simulink subsystem "PROPAGATOR"  (R2025b)
settings: Solver=VariableStepAuto  StartTime=0.0  StopTime=10.0  RelTol=1e-3
model mask{Parameter10=, Parameter11=, Parameter12=, Parameter13=, Parameter14=, Parameter4=, Parameter5=, Parameter6=, Parameter7=, quatConv=q4 (scalar last), forcesFrame=Inertial, r0=0, v0=0, att0=0, omg0=0, Parameter8=, Parameter9=}
  mask prompts: Parameter10 "State: 13x1 column vector, contains [inertial position; inertial velocity; inertial to body attitude; body to inertial angular velocity], in SI units"; Parameter11 "Force: 3x1 column vector, applied in the vehicle's CoG, in N"; Parameter12 "Torque: 3x1 column vector, applied in the vehicle's CoG, in Nm"; Parameter13 "Mass: 1x1 scalar, total mass of the vehicle, in kg"; Parameter14 "Inertia: 3x3 matrix, inertia tensor of the vehicle, in kgm2"; Parameter4 "Initial position: 3x1 column vector, inertial frame"; Parameter5 "Initial velocity: 3x1 column vector, inertial frame"; Parameter6 "Initial attitude: 4x1 column vector, rotation quaternion from inertial to body"; Parameter7 "Initial angular velocity: 3x1 column vector, angular rates in body frame w.r.t inertial frame"; quatConv "Quaternion convention"; forcesFrame "Forces reference frame"; r0 "Initial position [m]"; v0 "Initial velocity [ms-1]"; att0 "Initial attitude from inertial to body [-]"; omg0 "Initial angular velocity [rads-1]"; Parameter8 "Quaternion convention: Position of the scalar term"; Parameter9 "Forces reference frame: Forces in inertial frame or body frame"
libraries: aerolibutil x2, sharedutil x1, matrix_library x1
settings Model: Creator=antoniohernandez-rodiciomateos  LastModifiedBy=antoniohernandez-rodiciomateos

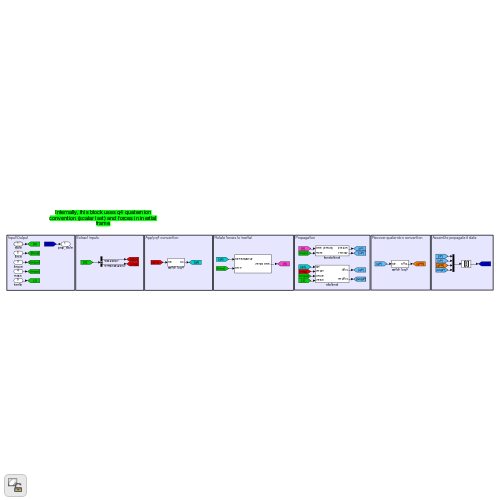
[thumbnail: Simulink's stored preview of the top-level diagram]
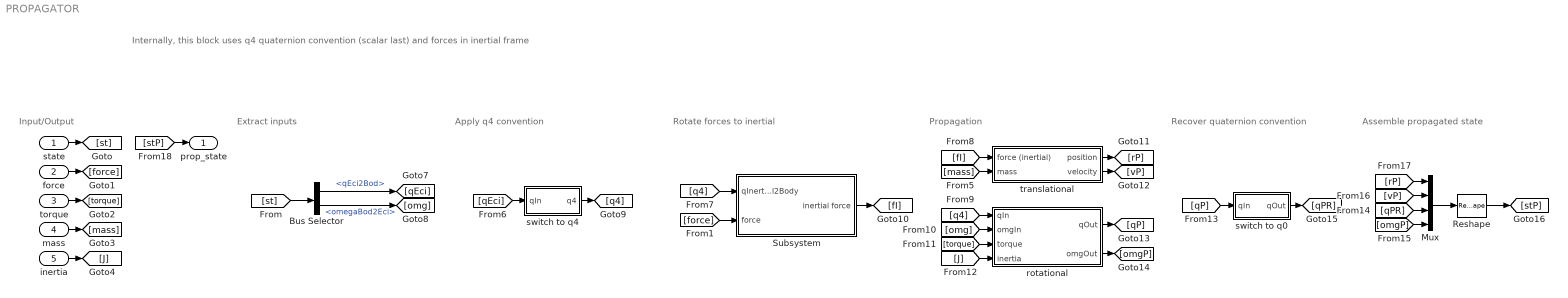
== system PROPAGATOR ==
  note: Input/Output
  note: Internally, this block uses q4 quaternion convention (scalar last) and forces in inertial frame
  note: Extract inputs
  note: Apply q4 convention
  note: Rotate forces to inertial
  note: Propagation
  note: Recover quaternion convention
  note: Assemble propagated state
  state : Inport  OutDataTypeStr=Bus: state_bus  PortDimensions=[13 1]
  force : Inport  Port=2  PortDimensions=[3 1]
  torque : Inport  Port=3  PortDimensions=[3 1]
  mass : Inport  Port=4  PortDimensions=[1 1]
  inertia : Inport  Port=5  PortDimensions=[3 3]
  Bus Selector : BusSelector  OutputSignals=qEci2Bod,omegaBod2Eci
  Mux : Mux
  Reshape : Reshape  OutputDimensionality=Column vector (2-D)
  Subsystem : Subsystem
  rotational : Subsystem
  switch to q0 : Subsystem
  switch to q4 : Subsystem
  translational : Subsystem
  prop_state : Outport  PortDimensions=[13 1]
  wires:
  state/1 -> [st]
  force/1 -> [force]
  torque/1 -> [torque]
  inertia/1 -> [J]
  mass/1 -> [mass]
  [st] -> Bus Selector/1
  Bus Selector/1 -> [qEci]  "<qEci2Bod>"
  Bus Selector/2 -> [omg]  "<omegaBod2Eci>"
  [q4] -> Subsystem/1(qInertial2Body)
  [force] -> Subsystem/2(force)
  [mass] -> translational/2(mass)
  Subsystem/1(inertial force) -> [fI]
  [fI] -> translational/1(force (inertial))
  [q4] -> rotational/1(qIn)
  [omg] -> rotational/2(omgIn)
  [torque] -> rotational/3(torque)
  [J] -> rotational/4(inertia)
  translational/1(position) -> [rP]
  translational/2(velocity) -> [vP]
  rotational/1(qOut) -> [qP]
  rotational/2(omgOut) -> [omgP]
  [qEci] -> switch to q4/1(qIn)
  switch to q4/1(q4) -> [q4]
  [qP] -> switch to q0/1(qIn)
  switch to q0/1(qOut) -> [qPR]
  [qPR] -> Mux/3
  [omgP] -> Mux/4
  [vP] -> Mux/2
  [rP] -> Mux/1
  [stP] -> prop_state/1
  Mux/1 -> Reshape/1
  Reshape/1 -> [stP]

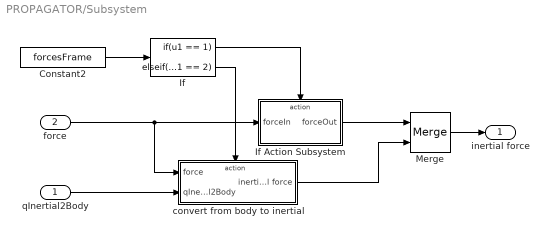
== system PROPAGATOR/Subsystem ==
  qInertial2Body : Inport  PortDimensions=[4 1]
  force : Inport  Port=2  PortDimensions=[3 1]
  Constant2 : Constant  Value=forcesFrame
  If : If  IfExpression=u1 == 1  ElseIfExpressions=u1 == 2  ShowElse=off
  If Action Subsystem : Subsystem  TreatAsAtomicUnit=on
  Merge : Merge
  convert from body to inertial : Subsystem  TreatAsAtomicUnit=on
  inertial force : Outport  PortDimensions=[3 1]
  wires:
  convert from body to inertial/1(inertial force) -> Merge/2
  If/1 -> If Action Subsystem/Action
  If Action Subsystem/1(forceOut) -> Merge/1
  force/1 -> convert from body to inertial/1(force), If Action Subsystem/1(forceIn)
  If/2 -> convert from body to inertial/Action
  Constant2/1 -> If/1
  Merge/1 -> inertial force/1
  qInertial2Body/1 -> convert from body to inertial/2(qInertial2Body)

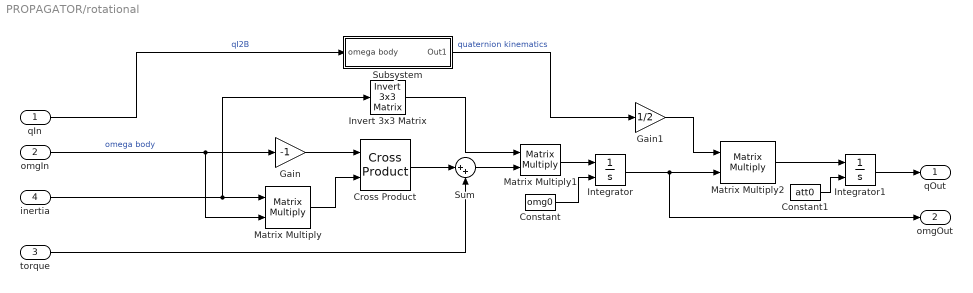
== system PROPAGATOR/rotational ==
  qIn : Inport  PortDimensions=[4 1]
  omgIn : Inport  Port=2  PortDimensions=[3 1]
  torque : Inport  Port=3  PortDimensions=[3 1]
  inertia : Inport  Port=4  PortDimensions=[3 3]
  Constant : Constant  Value=omg0
  Constant1 : Constant  Value=att0
  Cross Product : matrix_library/Cross Product
  Gain : Gain  Gain=-1
  Gain1 : Gain  Gain=1/2
  Integrator : Integrator  InitialConditionSource=external
  Integrator1 : Integrator  InitialConditionSource=external
  Invert 3x3 Matrix : aerolibutil/Invert  3x3 Matrix
  Matrix Multiply : Product  Multiplication=Matrix(*)
  Matrix Multiply1 : Product  Multiplication=Matrix(*)
  Matrix Multiply2 : Product  Multiplication=Matrix(*)
  Subsystem : Subsystem
  Sum : Sum  Inputs=|++
  qOut : Outport  PortDimensions=[4 1]
  omgOut : Outport  Port=2  PortDimensions=[3 1]
  wires:
  inertia/1 -> Invert 3x3 Matrix/1, Matrix Multiply/1
  Matrix Multiply/1 -> Cross Product/2
  omgIn/1 -> Gain/1, Matrix Multiply/2  "omega body"
  Gain/1 -> Cross Product/1
  Cross Product/1 -> Sum/1
  torque/1 -> Sum/2
  Sum/1 -> Matrix Multiply1/2
  Invert 3x3 Matrix/1 -> Matrix Multiply1/1
  Matrix Multiply1/1 -> Integrator/1
  Constant/1 -> Integrator/2
  qIn/1 -> Subsystem/1(omega body)  "qI2B"
  Subsystem/1(Out1) -> Gain1/1  "quaternion kinematics"
  Gain1/1 -> Matrix Multiply2/1
  Integrator/1 -> omgOut/1, Matrix Multiply2/2
  Integrator1/1 -> qOut/1
  Matrix Multiply2/1 -> Integrator1/1
  Constant1/1 -> Integrator1/2

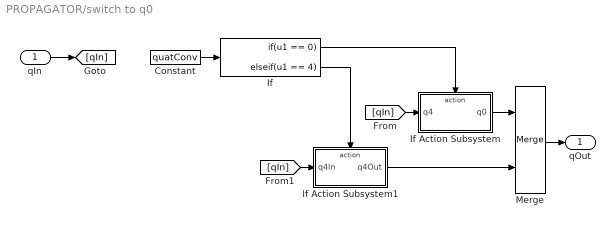
== system PROPAGATOR/switch to q0 ==
  qIn : Inport  PortDimensions=[4 1]
  Constant : Constant  Value=quatConv
  If : If  IfExpression=u1 == 0  ElseIfExpressions=u1 == 4  ShowElse=off
  If Action Subsystem : Subsystem  TreatAsAtomicUnit=on
  If Action Subsystem1 : Subsystem  TreatAsAtomicUnit=on
  Merge : Merge
  qOut : Outport  PortDimensions=[4 1]
  wires:
  If/1 -> If Action Subsystem/Action
  Merge/1 -> qOut/1
  Constant/1 -> If/1
  [qIn] -> If Action Subsystem/1(q4)
  If Action Subsystem1/1(q4Out) -> Merge/2
  [qIn] -> If Action Subsystem1/1(q4In)
  If Action Subsystem/1(q0) -> Merge/1
  If/2 -> If Action Subsystem1/Action
  qIn/1 -> [qIn]

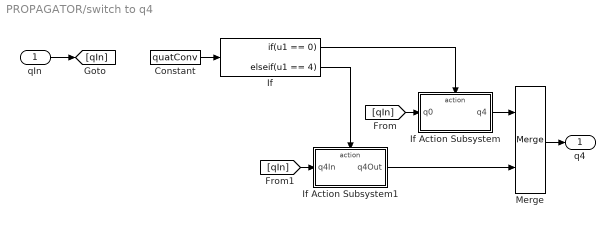
== system PROPAGATOR/switch to q4 ==
  qIn : Inport  PortDimensions=[4 1]
  Constant : Constant  Value=quatConv
  If : If  IfExpression=u1 == 0  ElseIfExpressions=u1 == 4  ShowElse=off
  If Action Subsystem : Subsystem  TreatAsAtomicUnit=on
  If Action Subsystem1 : Subsystem  TreatAsAtomicUnit=on
  Merge : Merge
  q4 : Outport  PortDimensions=[4 1]
  wires:
  If/1 -> If Action Subsystem/Action
  Merge/1 -> q4/1
  Constant/1 -> If/1
  [qIn] -> If Action Subsystem/1(q0)
  If Action Subsystem1/1(q4Out) -> Merge/2
  [qIn] -> If Action Subsystem1/1(q4In)
  If Action Subsystem/1(q4) -> Merge/1
  If/2 -> If Action Subsystem1/Action
  qIn/1 -> [qIn]

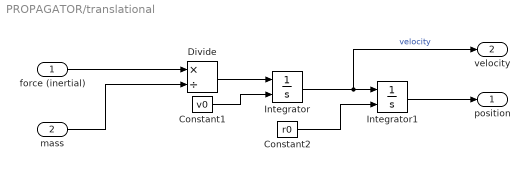
== system PROPAGATOR/translational ==
  force (inertial) : Inport  PortDimensions=[3 1]
  mass : Inport  Port=2  PortDimensions=[1 1]
  Constant1 : Constant  Value=v0
  Constant2 : Constant  Value=r0
  Divide : Product  Inputs=*/
  Integrator : Integrator  InitialConditionSource=external
  Integrator1 : Integrator  InitialConditionSource=external
  position : Outport  PortDimensions=[3 1]
  velocity : Outport  Port=2  PortDimensions=[3 1]
  wires:
  mass/1 -> Divide/2
  Constant1/1 -> Integrator/2
  Constant2/1 -> Integrator1/2
  Divide/1 -> Integrator/1
  Integrator1/1 -> position/1
  force (inertial)/1 -> Divide/1
  Integrator/1 -> velocity/1, Integrator1/1  "velocity"

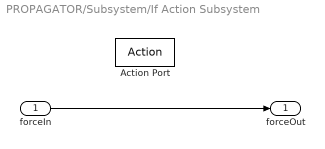
== system PROPAGATOR/Subsystem/If Action Subsystem ==
  forceIn : Inport  PortDimensions=[3 1]
  Action Port : ActionPort
  forceOut : Outport  PortDimensions=[3 1]
  wires:
  forceIn/1 -> forceOut/1

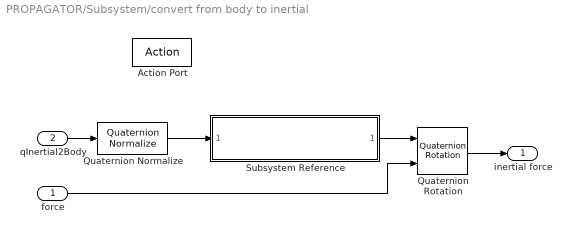
== system PROPAGATOR/Subsystem/convert from body to inertial ==
  force : Inport
  qInertial2Body : Inport  Port=2
  Action Port : ActionPort
  Quaternion Normalize : sharedutil/Quaternion Normalize  aMode=aMode
  Quaternion Rotation : aerolibutil/Quaternion Rotation
  Subsystem Reference : Subsystem  ReferencedSubsystem=quatConventionConverter  conversion=q4 to q0
  inertial force : Outport
  wires:
  force/1 -> Quaternion Rotation/2
  qInertial2Body/1 -> Quaternion Normalize/1
  Quaternion Normalize/1 -> Subsystem Reference/1
  Subsystem Reference/1 -> Quaternion Rotation/1
  Quaternion Rotation/1 -> inertial force/1

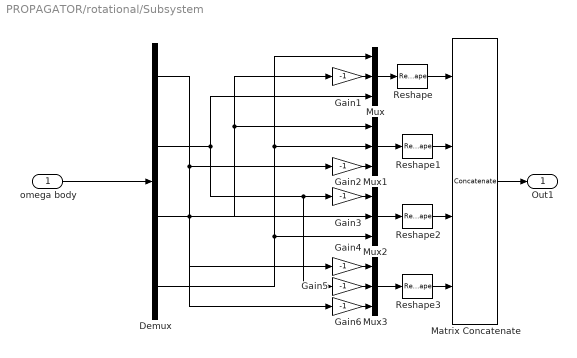
== system PROPAGATOR/rotational/Subsystem ==
  omega body : Inport  PortDimensions=[4 1]
  Demux : Demux
  Gain{1..6} (6 alike) : Gain  Gain=-1
  Matrix Concatenate : Concatenate  NumInputs=4  Mode=Multidimensional array
  Mux{,1..3} (4 alike) : Mux  Inputs=3
  Reshape{,1..3} (4 alike) : Reshape  OutputDimensionality=Row vector (2-D)
  Out1 : Outport  PortDimensions=[4 3]
  wires:
  omega body/1 -> Demux/1
  Mux/1 -> Reshape/1
  Reshape1/1 -> Matrix Concatenate/2
  Mux3/1 -> Reshape3/1
  Matrix Concatenate/1 -> Out1/1
  Reshape2/1 -> Matrix Concatenate/3
  Gain2/1 -> Mux1/3
  Gain5/1 -> Mux3/2
  Reshape3/1 -> Matrix Concatenate/4
  Mux2/1 -> Reshape2/1
  Demux/2 -> Gain5/1, Gain3/1, Mux/3
  Gain3/1 -> Mux2/1
  Demux/4 -> Mux2/3, Mux1/2, Mux/1
  Gain4/1 -> Mux3/1
  Mux1/1 -> Reshape1/1
  Gain1/1 -> Mux/2
  Gain6/1 -> Mux3/3
  Demux/1 -> Gain4/1, Mux2/2, Gain2/1
  Reshape/1 -> Matrix Concatenate/1
  Demux/3 -> Gain6/1, Mux1/1, Gain1/1

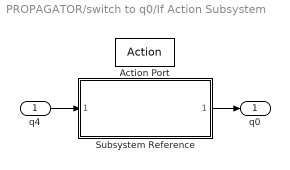
== system PROPAGATOR/switch to q0/If Action Subsystem ==
  q4 : Inport
  Action Port : ActionPort
  Subsystem Reference : Subsystem  ReferencedSubsystem=quatConventionConverter  conversion=q4 to q0
  q0 : Outport
  wires:
  q4/1 -> Subsystem Reference/1
  Subsystem Reference/1 -> q0/1

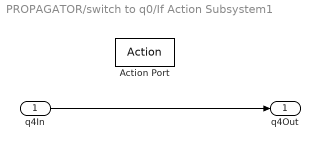
== system PROPAGATOR/switch to q0/If Action Subsystem1 ==
  q4In : Inport
  Action Port : ActionPort
  q4Out : Outport
  wires:
  q4In/1 -> q4Out/1

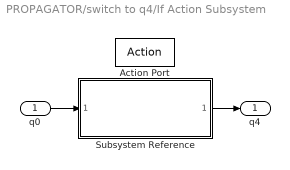
== system PROPAGATOR/switch to q4/If Action Subsystem ==
  q0 : Inport
  Action Port : ActionPort
  Subsystem Reference : Subsystem  ReferencedSubsystem=quatConventionConverter  conversion=q0 to q4
  q4 : Outport
  wires:
  q0/1 -> Subsystem Reference/1
  Subsystem Reference/1 -> q4/1

== system PROPAGATOR/switch to q4/If Action Subsystem1 ==
  q4In : Inport
  Action Port : ActionPort
  q4Out : Outport
  wires:
  q4In/1 -> q4Out/1
